simulink model "quarter_model_nonlin_R2018a"  (R2018a)
settings: Solver=VariableStepAuto  StartTime=0.0  StopTime=20  RelTol=1e-3
values from neighbouring files (symbols this model uses):
  b = 2e3    (= 2000)    [quarter_model_basic_script.m]    (also in quarter_model_nonlin_script.m)
  k2 = 2.09e4    (= 20900)    [quarter_model_basic_script.m]    (also in quarter_model_nonlin_script.m)
  m1 = 31    [quarter_model_basic_script.m]    (also in quarter_model_nonlin_script.m)
  m2 = 350    [quarter_model_basic_script.m]    (also in quarter_model_nonlin_script.m)
libraries: simulink x2
settings Model: Creator=kjartan  LastModifiedBy=kjartan
settings DataIOCC: ReturnWorkspaceOutputs=on
settings SFSimCC: SimUseLocalCustomCode=on
settings RTWCC: RTWUseLocalCustomCode=on

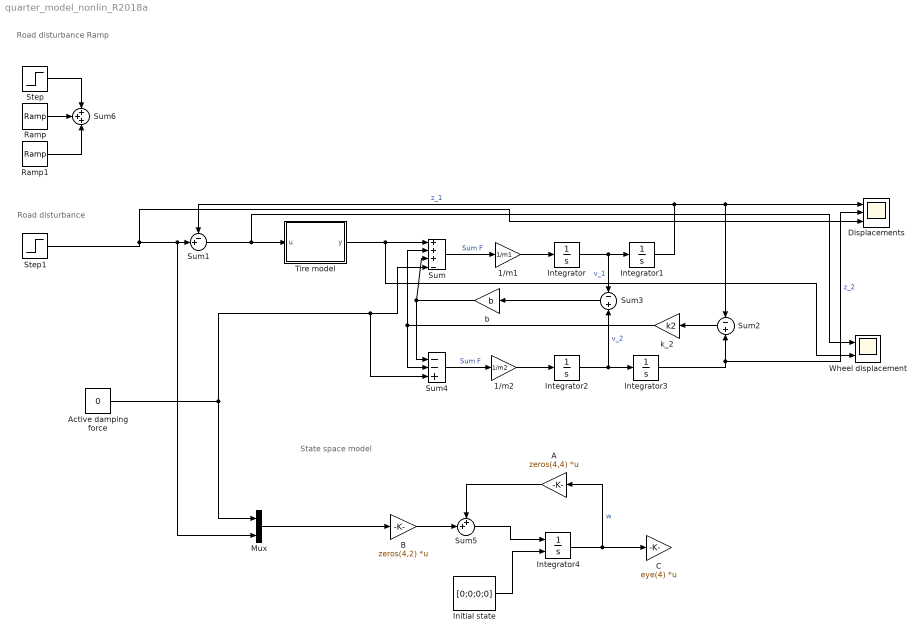
== system quarter_model_nonlin_R2018a ==
  note: Road disturbance
  note: Road disturbance
      | Ramp
  note: State space model
  1/m1 : Gain  Gain=1/m1
  1/m2 : Gain  Gain=1/m2
  A : Gain  Gain=zeros(4,4)  Multiplication=Matrix(K*u) (u vector)
  Active damping force : Constant  Value=0  OutDataTypeStr=Inherit: Inherit via back propagation
  B : Gain  Gain=zeros(4,2)  Multiplication=Matrix(K*u)
  C : Gain  Gain=eye(4)  Multiplication=Matrix(K*u) (u vector)
  Displacements : Scope  NumInputPorts=3
  Initial state : Constant  Value=[0;0;0;0]
  Integrator{,1..3} (4 alike) : Integrator
  Integrator4 : Integrator  InitialConditionSource=external
  Mux : Mux  Inputs=2
  Ramp : simulink/Sources/Ramp  slope=1  start=1  InitialOutput=0
  Ramp1 : simulink/Sources/Ramp  slope=-1  start=1.2  InitialOutput=0
  Step : Step  Time=1.2  After=-0.2  SampleTime=0
  Step1 : Step  After=0.1  SampleTime=0
  Sum : Sum  Inputs=+++-
  Sum1 : Sum  Inputs=-+|
  Sum2 : Sum  Inputs=-|+
  Sum3 : Sum  Inputs=-|+
  Sum4 : Sum  Inputs=--+
  Sum5 : Sum  Inputs=++|
  Sum6 : Sum  Inputs=+++
  Tire model : MATLAB Function  TreatAsAtomicUnit=on
  Wheel displacement : Scope  NumInputPorts=2
  b : Gain  Gain=b
  k_2 : Gain  Gain=k2
  wires:
  Integrator/1 -> Sum3/1, Integrator1/1  "v_1"
  Integrator1/1 -> Sum1/1, Sum2/1, Displacements/1  "z_1"
  Integrator2/1 -> Integrator3/1, Sum3/2  "v_2"
  Integrator3/1 -> Sum2/2, Displacements/2  "z_2"
  1/m2/1 -> Integrator2/1
  1/m1/1 -> Integrator/1
  Step1/1 -> Displacements/3, Mux/2, Sum1/2
  Sum3/1 -> b/1
  Tire model/1(y) -> Wheel displacement/2, Sum/1
  b/1 -> Sum4/1, Sum/3
  Sum2/1 -> k_2/1
  k_2/1 -> Sum/2, Sum4/2
  Sum/1 -> 1/m1/1  "Sum F"
  Active damping force/1 -> Mux/1, Sum4/3, Sum/4
  Sum4/1 -> 1/m2/1  "Sum F"
  Initial state/1 -> Integrator4/2
  B/1 -> Sum5/2
  Sum5/1 -> Integrator4/1
  Integrator4/1 -> A/1, C/1  "w"
  A/1 -> Sum5/1
  Mux/1 -> B/1
  Sum1/1 -> Wheel displacement/1, Tire model/1(u)
  Ramp/1 -> Sum6/2
  Ramp1/1 -> Sum6/3
  Step/1 -> Sum6/1

== matlab function quarter_model_nonlin_R2018a/Tire model ==
  data: u input; y output
function y = fcn(u)
  k1 = 1.08e5;
  tire_spring_ll = -0.0346;
  tire_spring_ul = 0.1;
  if (u < tire_spring_ll)
      y = k1*tire_spring_ll;
  elseif (u > tire_spring_ul)
      y = k1*tire_spring_ul + 10*k1*(u-tire_spring_ul);
  else
      y = k1*u;
  end
end
